simulink model "Regler"  (R2015b)
settings: Solver=VariableStepAuto  StartTime=0.0  StopTime=20  RelTol=1e-3
settings Model: Creator=danielhauer  LastModifiedBy=Christoph Zech

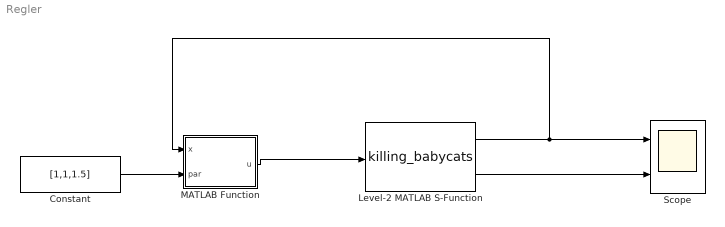
== system Regler ==
  Constant : Constant  Value=[1,1,1.5]
  Level-2 MATLAB S-Function : M-S-Function  FunctionName=killing_babycats  Parameters=[4,0.5]
  MATLAB Function : MATLAB Function  TreatAsAtomicUnit=on
  Scope : Scope  NumInputPorts=2
  wires:
  MATLAB Function/1(u) -> Level-2 MATLAB S-Function/1
  Level-2 MATLAB S-Function/1 -> MATLAB Function/1(x), Scope/1
  Level-2 MATLAB S-Function/2 -> Scope/2
  Constant/1 -> MATLAB Function/2(par)

== matlab function Regler/MATLAB Function ==
  data: u output; x input; par input
function u = Regler(x,par)

%c1=0.5;
%c2=10;

c1 = 0.5;
c2 = 10;
x1_soll=1.5;

x1=x(1);
x2=x(2);



alpha = 1 - c1*(x1-x1_soll)/x1;
dalphadx = -c1*x1_soll/x1^2;
g2 = x2;
f2 = x2-x1*x2;
g1 = x1;
f1 = -x1;

%alte Lösung (falsch, aber funktioniert)
%u=1/x2*(x2*x1-x2-c1*(x2+c1*(x1-x1_soll)/x1-1));
%u = 1/g2 * (-f2 - c2*(x2-alpha));

%Lösungen stimmen eh überein hab ich vorher gemerkt ^^
%Lösung laut Skript:
%u = 1/g2 * ( -f2 + dalphadx*(f1+g1*x2) - (x1-x1_soll)*x1 - c2*(x2-alpha));
%Meine Lösung
u = 1/g2 * ( -f2 + dalphadx*(f1+g1*x2) - (x1-x1_soll)*g1 - c2*(x2-alpha));


end
